simulink model "set_point"  (R2020a)
settings: Solver=VariableStepAuto  StartTime=0.0  StopTime=30  RelTol=1e-3
undefined symbols (not defined in the file): r
settings Model: Creator=Ferran  LastModifiedBy=Ferran

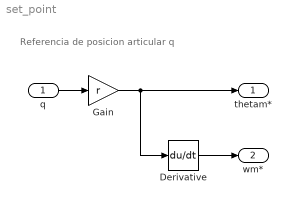
== system set_point ==
  note: Referencia de posicion articular q
  q : Inport
  Derivative : Derivative
  Gain : Gain  Gain=r
  thetam* : Outport
  wm* : Outport  Port=2
  wires:
  Gain/1 -> thetam*/1, Derivative/1
  Derivative/1 -> wm*/1
  q/1 -> Gain/1
